simulink model "verify_voltrip_3series"  (R2016a)
settings: Solver=ode4  StartTime=0.0  StopTime=Tmax  FixedStep=Ts  RelTol=1e-3
values from neighbouring files (symbols this model uses):
  Cdc = 50e-6    (= 5e-05)    [pemd_simulink_base.m]
  Lload = Xload/wout    [pemd_simulink_base.m]
  ma = 0.9    [optim_v1.m]    (also in pemd_simulink_base.m = 0.8)
  phase = [0 (k-1)*10 (k-1)*20 (k-1)*30]    [pemd_simulink_base.m]
  Rin = 10    [pemd_simulink_base.m]
  Rload = Zload*pf    [pemd_simulink_base.m]
  Ts = 1e-6    (= 1e-06)    [pemd_simulink_base.m]
  Tth = 0.04    [pemd_simulink_base.m]
  Vin = Vdc + Rin*(Ptotal/Vdc)    (= 697.604412924)    [pemd_simulink_base.m]
  wout = 2*pi*fout    (= 314.159265359)    [pemd_simulink_base.m]
libraries: powerlib x41, powerlib_meascontrol x16, simulink x8
settings Model: Creator=ugurm  LastModifiedBy=mesutto
settings DataIOCC: LimitDataPoints=on  SaveFormat=Array
settings DebuggingCC: UnderspecifiedInitializationDetection=Classic  MergeDetectMultiDrivingBlocksExec=none  SolverPrmCheckMsg=warning  StateNameClashWarn=warning
settings HardwareCC: ProdBitPerPointer=32  ProdLargestAtomicFloat=None  ProdIntDivRoundTo=Undefined  ProdEndianess=Unspecified  ProdWordSize=32  ProdHWDeviceType=32-bit Generic
settings ModelReferenceCC: PropagateSignalLabelsOutOfModel=off
settings ConfigComp: CovModelRefEnable=Off

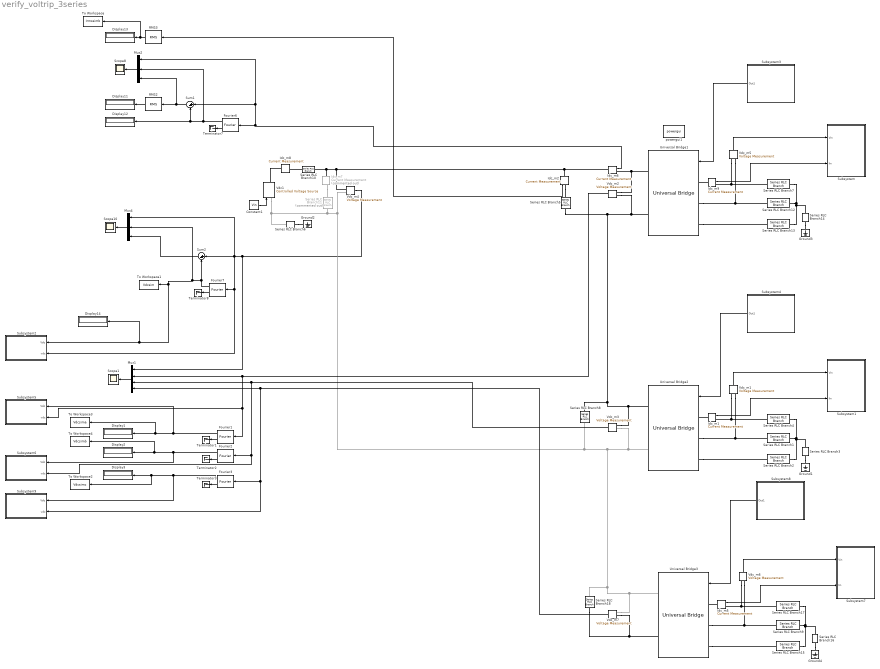
== system verify_voltrip_3series ==
  Constant1 : Constant  Value=Vin
  Display{1..3,11..14} (7 alike) : Display
  Fourier{1..3,7} (4 alike) : powerlib_meascontrol/Measurements/Fourier  Freq=fout  n=0  InInit=[0, 0]  Ts=Ts
  Fourier6 : powerlib_meascontrol/Measurements/Fourier  Freq=fout  n=0  InInit=[20, 0]  Ts=Ts
  Ground{1..4} (4 alike) : powerlib/Elements/Ground  LConnTagsString=a
  Idc_m{1..2,5..6,8..9} (6 alike) : powerlib/Measurements/Current Measurement  PhasorSimulation=off  OutputType=Complex  PSBequivalent=0
  Idc_m7 : powerlib/Measurements/Current Measurement  Commented=on  PhasorSimulation=off  OutputType=Complex  PSBequivalent=0
  Mux1 : Mux
  Mux2 : Mux  Inputs=3
  Mux4 : Mux  Inputs=3
  RMS2 : powerlib_meascontrol/Measurements/RMS  TrueRMS=on  Freq=fout  RMSInit=10  Ts=Ts
  RMS3 : powerlib_meascontrol/Measurements/RMS  TrueRMS=on  Freq=fout  RMSInit=10  Ts=Ts
  Scope1 : Scope
  Scope10 : Scope
  Scope8 : Scope
  Series RLC Branch{1..2,4,7,9,12..13,15,17} (9 alike) : powerlib/Elements/Series RLC Branch  LConnTagsString=__new0  RConnTagsString=__new0  BranchType=RL  Resistance=Rload  Inductance=Lload  SetiL0=off  InitialCurrent=0  Capacitance=1e-6  Setx0=off  InitialVoltage=0  Measurements=None
  Series RLC Branch10 : powerlib/Elements/Series RLC Branch  LConnTagsString=__new0  RConnTagsString=__new0  BranchType=R  Resistance=Rin  Inductance=Lload  SetiL0=off  InitialCurrent=0  Capacitance=1e-6  Setx0=off  InitialVoltage=0  Measurements=None
  Series RLC Branch11 : powerlib/Elements/Series RLC Branch  Commented=on  LConnTagsString=__new0  RConnTagsString=__new0  BranchType=C  Resistance=1e12  Inductance=Lload  SetiL0=off  InitialCurrent=0  Capacitance=Cdc  Setx0=off  InitialVoltage=0  Measurements=None
  Series RLC Branch{3,6,14,16} (4 alike) : powerlib/Elements/Series RLC Branch  LConnTagsString=__new0  RConnTagsString=__new0  BranchType=R  Resistance=1e12  Inductance=Lload  SetiL0=off  InitialCurrent=0  Capacitance=1e-6  Setx0=off  InitialVoltage=0  Measurements=None
  Series RLC Branch18 : powerlib/Elements/Series RLC Branch  LConnTagsString=__new0  RConnTagsString=__new0  BranchType=C  Resistance=1e12  Inductance=Lload  SetiL0=off  InitialCurrent=0  Capacitance=Cdc  Setx0=off  InitialVoltage=0  Measurements=None
  Series RLC Branch5 : powerlib/Elements/Series RLC Branch  LConnTagsString=__new0  RConnTagsString=__new0  BranchType=C  Resistance=1e12  Inductance=Lload  SetiL0=off  InitialCurrent=0  Capacitance=Cdc  Setx0=off  InitialVoltage=0  Measurements=None
  Series RLC Branch8 : powerlib/Elements/Series RLC Branch  LConnTagsString=__new0  RConnTagsString=__new0  BranchType=C  Resistance=1e12  Inductance=Lload  SetiL0=off  InitialCurrent=0  Capacitance=Cdc  Setx0=off  InitialVoltage=0  Measurements=None
  Subsystem : Subsystem
  Subsystem1 : Subsystem
  Subsystem2 : Subsystem
  Subsystem3 : Subsystem
  Subsystem4 : Subsystem
  Subsystem5 : Subsystem
  Subsystem6 : Subsystem
  Subsystem7 : Subsystem
  Subsystem8 : Subsystem
  Subsystem9 : Subsystem
  Sum1 : Sum  Inputs=|+-
  Sum2 : Sum  Inputs=|+-
  Terminator{1..3,7..8} (5 alike) : Terminator
  To Workspace : ToWorkspace  VariableName=Irmssimb  SampleTime=-1
  To Workspace1 : ToWorkspace  VariableName=Vdcsim  SampleTime=-1
  To Workspace2 : ToWorkspace  VariableName=Vdcsimc  SampleTime=-1
  To Workspace3 : ToWorkspace  VariableName=Vdcsima  SampleTime=-1
  To Workspace4 : ToWorkspace  VariableName=Vdcsimb  SampleTime=-1
  Universal Bridge1 : powerlib/Power Electronics/Universal Bridge  Arms=3  SnubberResistance=1e5  SnubberCapacitance=inf  Device=IGBT / Diodes  Ron=1e-6  Lon=0  ForwardVoltages="[  0  0  ]"  ForwardVoltage=0  GTOparameters=[ 10e-6 , 20e-6 ]  IGBTparameters=[ 1e-6 , 2e-6 ]  Measurements=None  Measurements_2=None  converterType=Rectifier
  Universal Bridge2 : powerlib/Power Electronics/Universal Bridge  Arms=3  SnubberResistance=1e5  SnubberCapacitance=inf  Device=IGBT / Diodes  Ron=1e-6  Lon=0  ForwardVoltages="[  0  0  ]"  ForwardVoltage=0  GTOparameters=[ 10e-6 , 20e-6 ]  IGBTparameters=[ 1e-6 , 2e-6 ]  Measurements=None  Measurements_2=None  converterType=Rectifier
  Universal Bridge3 : powerlib/Power Electronics/Universal Bridge  Arms=3  SnubberResistance=1e5  SnubberCapacitance=inf  Device=IGBT / Diodes  Ron=1e-6  Lon=0  ForwardVoltages="[  0  0  ]"  ForwardVoltage=0  GTOparameters=[ 10e-6 , 20e-6 ]  IGBTparameters=[ 1e-6 , 2e-6 ]  Measurements=None  Measurements_2=None  converterType=Rectifier
  Vdc1 : powerlib/Electrical Sources/Controlled Voltage Source  Initialize=off  Source_Type=DC  Amplitude=200  Phase=0  Frequency=0  Measurements=None
  Vdc_m{1..7} (7 alike) : powerlib/Measurements/Voltage Measurement  PhasorSimulation=off  OutputType=Complex  PSBequivalent=0
  powergui1 : powerlib/powergui  Priority=1  SimulationMode=Discrete  SolverType=Tustin  SampleTime=Ts  frequency=60  SPID=off  DisableSnubberDevices=off  DisableRonSwitches=off  DisableVfSwitches=off  SwTol=0  DisplayEquations=off  Interpol=off  ExternalGateDelay=off  methode=off  Ts=0  FunctionMessages=off  echomessages=off  HookPort=off  EnableUseOfTLC=off  x0status=blocks  frequencyindice=0  Pbase=100e6  ErrMax=1e-4  Iterations=50  UnitsV=kV  UnitsW=MW  buscounter=0  RestoreLinks=warning  ResistiveCurrentMeasurement=off  Frange=[0:2:500]  Ylog=off  Xlog=on  ShowGrid=off  save=off  variable=ZData  structure=idc  ZoomFFT=off  StartTime=0.1  cycles=20  DisplayStyle=5  fundamental=50  FreqAxis=off  MaxFrequency=20000  frequencyindicesteady=1  RmsSteady=1  display=off
  wires:
  Fourier6/2 -> Terminator7/1
  RMS2/1 -> Display11/1
  Fourier6/1 -> Mux2/2, Sum1/2, Display12/1
  Sum1/1 -> Mux2/3, RMS2/1
  Constant1/1 -> Vdc1/1
  Idc_m6/1 -> Sum1/1, Mux2/1, Fourier6/1
  Mux2/1 -> Scope8/1
  RMS3/1 -> To Workspace/1, Display13/1
  Fourier7/2 -> Terminator8/1
  Fourier7/1 -> Sum2/2, Mux4/2, Display14/1, Subsystem2/1(Vdc), To Workspace1/1
  Vdc_m4/1 -> Mux1/1, Mux4/1, Subsystem2/2(vdc), Fourier7/1, Sum2/1
  Mux4/1 -> Scope10/1
  Sum2/1 -> Mux4/3
  Subsystem3/1(Out1) -> Universal Bridge1/1
  Vdc_m5/1 -> Subsystem/1(Vin)
  Idc_m9/1 -> Subsystem/2(Iin)
  Subsystem4/1(Out1) -> Universal Bridge2/1
  Vdc_m1/1 -> Subsystem1/1(Vin)
  Idc_m1/1 -> Subsystem1/2(Iin)
  Fourier1/2 -> Terminator1/1
  Fourier1/1 -> Subsystem5/1(Vdc), To Workspace3/1, Display1/1
  Mux1/1 -> Scope1/1
  Fourier2/2 -> Terminator2/1
  Fourier2/1 -> Subsystem6/1(Vdc), Display2/1, To Workspace4/1
  Idc_m2/1 -> RMS3/1
  Subsystem8/1(Out1) -> Universal Bridge3/1
  Vdc_m6/1 -> Subsystem7/1(Vin)
  Idc_m5/1 -> Subsystem7/2(Iin)
  Fourier3/2 -> Terminator3/1
  Fourier3/1 -> Subsystem9/1(Vdc), To Workspace2/1, Display3/1
  Vdc_m2/1 -> Subsystem5/2(vdc), Fourier1/1, Mux1/2
  Vdc_m3/1 -> Subsystem6/2(vdc), Fourier2/1, Mux1/3
  Vdc_m7/1 -> Subsystem9/2(vdc), Fourier3/1, Mux1/4
  connections:
  Universal Bridge1/RConn1 -- Vdc_m2/LConn1 -- Idc_m6/RConn1
  Idc_m7/RConn1 -- Series RLC Branch11/LConn1
  Series RLC Branch6/RConn1 -- Ground2/LConn1
  Series RLC Branch10/RConn1 -- Idc_m8/RConn1
  Vdc1/RConn1 -- Idc_m8/LConn1
  Universal Bridge1/LConn3 -- Series RLC Branch13/LConn1
  Series RLC Branch12/LConn1 -- Universal Bridge1/LConn2 -- Vdc_m5/LConn2
  Vdc_m5/LConn1 -- Idc_m9/RConn1 -- Series RLC Branch7/LConn1
  Series RLC Branch12/RConn1 -- Series RLC Branch14/LConn1 -- Series RLC Branch13/RConn1 -- Series RLC Branch7/RConn1
  Series RLC Branch14/RConn1 -- Ground3/LConn1
  Idc_m9/LConn1 -- Universal Bridge1/LConn1
  Vdc_m1/LConn2 -- Universal Bridge2/LConn2 -- Series RLC Branch1/LConn1
  Vdc_m1/LConn1 -- Idc_m1/RConn1 -- Series RLC Branch4/LConn1
  Series RLC Branch2/RConn1 -- Series RLC Branch4/RConn1 -- Series RLC Branch1/RConn1 -- Series RLC Branch3/LConn1
  Idc_m1/LConn1 -- Universal Bridge2/LConn1
  Series RLC Branch3/RConn1 -- Ground1/LConn1
  Universal Bridge2/LConn3 -- Series RLC Branch2/LConn1
  Idc_m2/RConn1 -- Series RLC Branch5/LConn1
  Vdc_m4/LConn1 -- Idc_m6/LConn1 -- Idc_m2/LConn1 -- Series RLC Branch10/LConn1 -- Idc_m7/LConn1
  Series RLC Branch5/RConn1 -- Series RLC Branch8/LConn1 -- Vdc_m3/LConn1 -- Universal Bridge2/RConn1 -- Vdc_m2/LConn2 -- Universal Bridge1/RConn2
  Vdc_m6/LConn2 -- Universal Bridge3/LConn2 -- Series RLC Branch9/LConn1
  Vdc_m6/LConn1 -- Idc_m5/RConn1 -- Series RLC Branch17/LConn1
  Series RLC Branch15/RConn1 -- Series RLC Branch16/LConn1 -- Series RLC Branch17/RConn1 -- Series RLC Branch9/RConn1
  Universal Bridge3/LConn3 -- Series RLC Branch15/LConn1
  Idc_m5/LConn1 -- Universal Bridge3/LConn1
  Series RLC Branch16/RConn1 -- Ground4/LConn1
  Series RLC Branch11/RConn1 -- Series RLC Branch18/LConn1 -- Vdc_m7/LConn1 -- Universal Bridge3/RConn1 -- Vdc_m3/LConn2 -- Universal Bridge2/RConn2 -- Series RLC Branch8/RConn1 -- Vdc_m4/LConn2 -- Vdc1/LConn1 -- Series RLC Branch6/LConn1
  Vdc_m7/LConn2 -- Series RLC Branch18/RConn1 -- Universal Bridge3/RConn2

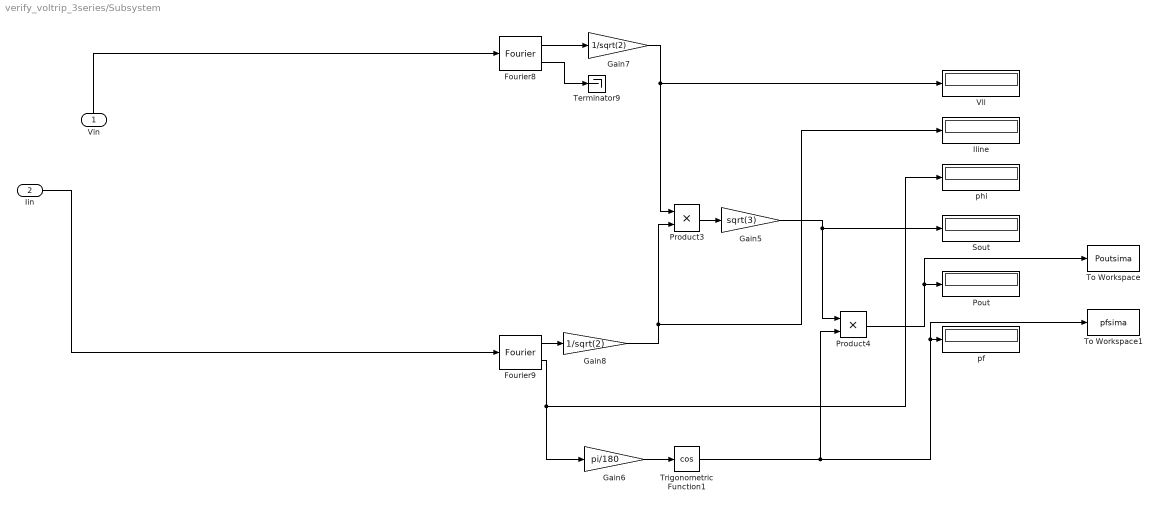
== system verify_voltrip_3series/Subsystem ==
  Vin : Inport
  Iin : Inport  Port=2
  Fourier8 : powerlib_meascontrol/Measurements/Fourier  Freq=fout  n=1  InInit=[0, 0]  Ts=Ts
  Fourier9 : powerlib_meascontrol/Measurements/Fourier  Freq=fout  n=1  InInit=[0, 0]  Ts=Ts
  Gain5 : Gain  Gain=sqrt(3)
  Gain6 : Gain  Gain=pi/180
  Gain7 : Gain  Gain=1/sqrt(2)
  Gain8 : Gain  Gain=1/sqrt(2)
  Iline : Display
  Pout : Display
  Product3 : Product
  Product4 : Product
  Sout : Display
      settings: Format=short_e
  Terminator9 : Terminator
  To Workspace : ToWorkspace  VariableName=Poutsima  SampleTime=-1
  To Workspace1 : ToWorkspace  VariableName=pfsima  SampleTime=-1
  Trigonometric Function1 : Trigonometry  Operator=cos
  Vll : Display
  pf : Display
  phi : Display
  wires:
  Gain6/1 -> Trigonometric Function1/1
  Gain8/1 -> Iline/1, Product3/2
  Gain5/1 -> Product4/1, Sout/1
  Trigonometric Function1/1 -> Product4/2, To Workspace1/1, pf/1
  Vin/1 -> Fourier8/1
  Iin/1 -> Fourier9/1
  Fourier8/2 -> Terminator9/1
  Fourier8/1 -> Gain7/1
  Product3/1 -> Gain5/1
  Gain7/1 -> Product3/1, Vll/1
  Product4/1 -> To Workspace/1, Pout/1
  Fourier9/2 -> Gain6/1, phi/1
  Fourier9/1 -> Gain8/1

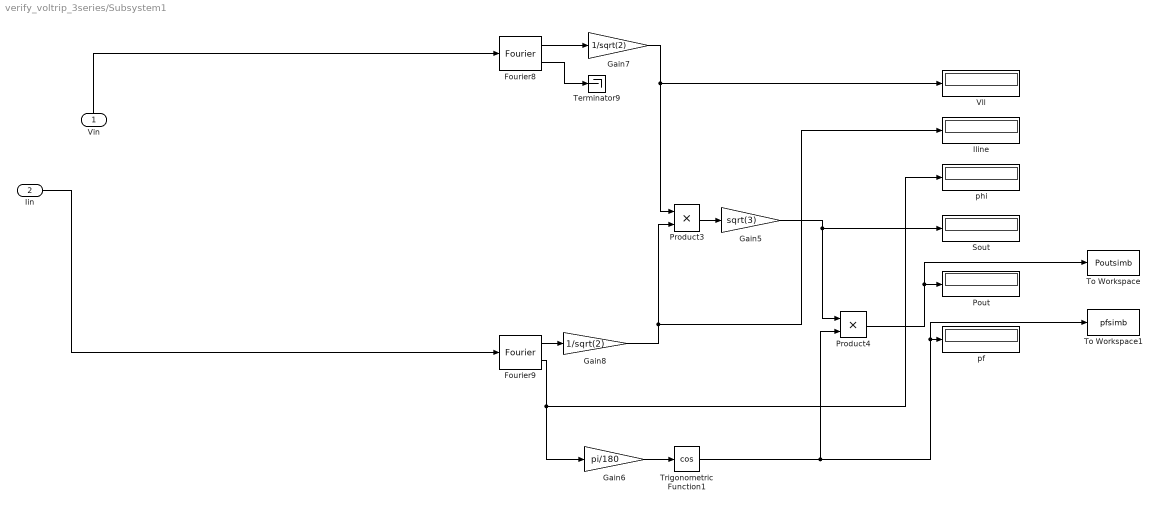
== system verify_voltrip_3series/Subsystem1 ==
  Vin : Inport
  Iin : Inport  Port=2
  Fourier8 : powerlib_meascontrol/Measurements/Fourier  Freq=fout  n=1  InInit=[0, 0]  Ts=Ts
  Fourier9 : powerlib_meascontrol/Measurements/Fourier  Freq=fout  n=1  InInit=[0, 0]  Ts=Ts
  Gain5 : Gain  Gain=sqrt(3)
  Gain6 : Gain  Gain=pi/180
  Gain7 : Gain  Gain=1/sqrt(2)
  Gain8 : Gain  Gain=1/sqrt(2)
  Iline : Display
  Pout : Display
  Product3 : Product
  Product4 : Product
  Sout : Display
      settings: Format=short_e
  Terminator9 : Terminator
  To Workspace : ToWorkspace  VariableName=Poutsimb  SampleTime=-1
  To Workspace1 : ToWorkspace  VariableName=pfsimb  SampleTime=-1
  Trigonometric Function1 : Trigonometry  Operator=cos
  Vll : Display
  pf : Display
  phi : Display
  wires:
  Gain6/1 -> Trigonometric Function1/1
  Gain8/1 -> Iline/1, Product3/2
  Gain5/1 -> Product4/1, Sout/1
  Trigonometric Function1/1 -> Product4/2, To Workspace1/1, pf/1
  Vin/1 -> Fourier8/1
  Iin/1 -> Fourier9/1
  Fourier8/2 -> Terminator9/1
  Fourier8/1 -> Gain7/1
  Product3/1 -> Gain5/1
  Gain7/1 -> Product3/1, Vll/1
  Product4/1 -> To Workspace/1, Pout/1
  Fourier9/2 -> Gain6/1, phi/1
  Fourier9/1 -> Gain8/1

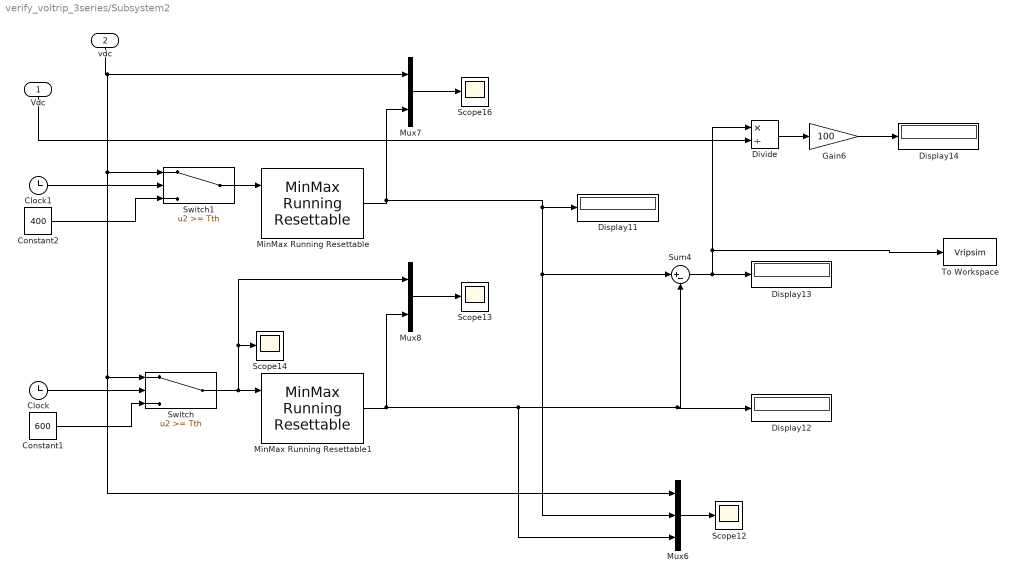
== system verify_voltrip_3series/Subsystem2 ==
  Vdc : Inport
  vdc : Inport  Port=2
  Clock : Clock
  Clock1 : Clock
  Constant1 : Constant  Value=600  SampleTime=Ts
  Constant2 : Constant  Value=400  SampleTime=Ts
  Display{11..14} (4 alike) : Display
  Divide : Product  Inputs=*/
  Gain6 : Gain  Gain=100
  MinMax Running Resettable : simulink/Math Operations/MinMax Running Resettable  Function=max  vinit=400
  MinMax Running Resettable1 : simulink/Math Operations/MinMax Running Resettable  Function=min  vinit=600
  Mux6 : Mux  Inputs=3
  Mux7 : Mux  Inputs=2
  Mux8 : Mux  Inputs=2
  Scope{12..14,16} (4 alike) : Scope
  Sum4 : Sum  Inputs=|+-
  Switch : Switch  Threshold=Tth
  Switch1 : Switch  Threshold=Tth
  To Workspace : ToWorkspace  VariableName=Vripsim  SampleTime=-1
  wires:
  MinMax Running Resettable/1 -> Display11/1, Mux6/2, Sum4/1, Mux7/2
  Clock/1 -> Switch/2
  Mux8/1 -> Scope13/1
  Gain6/1 -> Display14/1
  Constant1/1 -> Switch/3
  MinMax Running Resettable1/1 -> Mux6/3, Display12/1, Sum4/2, Mux8/2
  Mux7/1 -> Scope16/1
  Switch/1 -> Mux8/1, Scope14/1, MinMax Running Resettable1/1
  Divide/1 -> Gain6/1
  Mux6/1 -> Scope12/1
  Vdc/1 -> Divide/2
  vdc/1 -> Mux7/1, Switch1/1, Mux6/1, Switch/1
  Clock1/1 -> Switch1/2
  Constant2/1 -> Switch1/3
  Switch1/1 -> MinMax Running Resettable/1
  Sum4/1 -> To Workspace/1, Divide/1, Display13/1

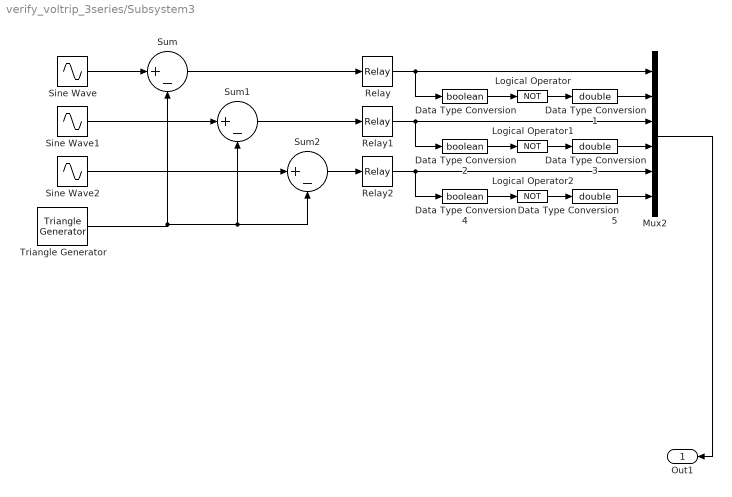
== system verify_voltrip_3series/Subsystem3 ==
  Data Type Conversion : DataTypeConversion  OutDataTypeStr=boolean
  Data Type Conversion1 : DataTypeConversion  OutDataTypeStr=double
  Data Type Conversion2 : DataTypeConversion  OutDataTypeStr=boolean
  Data Type Conversion3 : DataTypeConversion  OutDataTypeStr=double
  Data Type Conversion4 : DataTypeConversion  OutDataTypeStr=boolean
  Data Type Conversion5 : DataTypeConversion  OutDataTypeStr=double
  Logical Operator : Logic  Operator=NOT  AllPortsSameDT=off  OutDataTypeStr=boolean
  Logical Operator1 : Logic  Operator=NOT  AllPortsSameDT=off  OutDataTypeStr=boolean
  Logical Operator2 : Logic  Operator=NOT  AllPortsSameDT=off  OutDataTypeStr=boolean
  Mux2 : Mux  Inputs=6
  Relay : Relay
  Relay1 : Relay
  Relay2 : Relay
  Sine Wave : Sin  Amplitude=ma  Frequency=wout  SampleTime=0
  Sine Wave1 : Sin  Amplitude=ma  Frequency=wout  Phase=-2*pi/3  SampleTime=0
  Sine Wave2 : Sin  Amplitude=ma  Frequency=wout  Phase=2*pi/3  SampleTime=0
  Sum : Sum  Inputs=|+-
  Sum1 : Sum  Inputs=|+-
  Sum2 : Sum  Inputs=|+-
  Triangle Generator : powerlib_meascontrol/Pulse & Signal Generators/Triangle Generator  Freq=fsw  Phase=phase(1)  Ts=Ts
  Out1 : Outport
  wires:
  Logical Operator1/1 -> Data Type Conversion3/1
  Sum/1 -> Relay/1
  Triangle Generator/1 -> Sum1/2, Sum2/2, Sum/2
  Logical Operator/1 -> Data Type Conversion1/1
  Relay1/1 -> Data Type Conversion2/1, Mux2/3
  Logical Operator2/1 -> Data Type Conversion5/1
  Data Type Conversion4/1 -> Logical Operator2/1
  Data Type Conversion2/1 -> Logical Operator1/1
  Data Type Conversion5/1 -> Mux2/6
  Sine Wave2/1 -> Sum2/1
  Data Type Conversion3/1 -> Mux2/4
  Sum1/1 -> Relay1/1
  Relay2/1 -> Data Type Conversion4/1, Mux2/5
  Relay/1 -> Data Type Conversion/1, Mux2/1
  Mux2/1 -> Out1/1
  Data Type Conversion1/1 -> Mux2/2
  Sine Wave/1 -> Sum/1
  Sine Wave1/1 -> Sum1/1
  Data Type Conversion/1 -> Logical Operator/1
  Sum2/1 -> Relay2/1

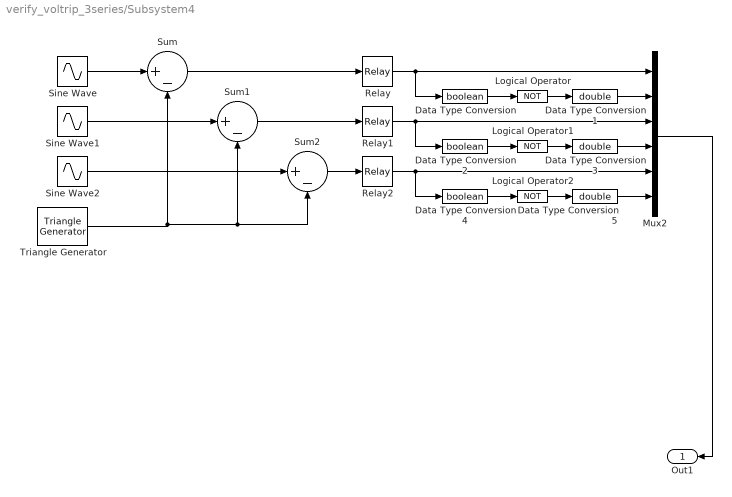
== system verify_voltrip_3series/Subsystem4 ==
  Data Type Conversion : DataTypeConversion  OutDataTypeStr=boolean
  Data Type Conversion1 : DataTypeConversion  OutDataTypeStr=double
  Data Type Conversion2 : DataTypeConversion  OutDataTypeStr=boolean
  Data Type Conversion3 : DataTypeConversion  OutDataTypeStr=double
  Data Type Conversion4 : DataTypeConversion  OutDataTypeStr=boolean
  Data Type Conversion5 : DataTypeConversion  OutDataTypeStr=double
  Logical Operator : Logic  Operator=NOT  AllPortsSameDT=off  OutDataTypeStr=boolean
  Logical Operator1 : Logic  Operator=NOT  AllPortsSameDT=off  OutDataTypeStr=boolean
  Logical Operator2 : Logic  Operator=NOT  AllPortsSameDT=off  OutDataTypeStr=boolean
  Mux2 : Mux  Inputs=6
  Relay : Relay
  Relay1 : Relay
  Relay2 : Relay
  Sine Wave : Sin  Amplitude=ma  Frequency=wout  SampleTime=0
  Sine Wave1 : Sin  Amplitude=ma  Frequency=wout  Phase=-2*pi/3  SampleTime=0
  Sine Wave2 : Sin  Amplitude=ma  Frequency=wout  Phase=2*pi/3  SampleTime=0
  Sum : Sum  Inputs=|+-
  Sum1 : Sum  Inputs=|+-
  Sum2 : Sum  Inputs=|+-
  Triangle Generator : powerlib_meascontrol/Pulse & Signal Generators/Triangle Generator  Freq=fsw  Phase=phase(2)  Ts=Ts
  Out1 : Outport
  wires:
  Logical Operator1/1 -> Data Type Conversion3/1
  Sum/1 -> Relay/1
  Triangle Generator/1 -> Sum1/2, Sum2/2, Sum/2
  Logical Operator/1 -> Data Type Conversion1/1
  Relay1/1 -> Data Type Conversion2/1, Mux2/3
  Logical Operator2/1 -> Data Type Conversion5/1
  Data Type Conversion4/1 -> Logical Operator2/1
  Data Type Conversion2/1 -> Logical Operator1/1
  Data Type Conversion5/1 -> Mux2/6
  Sine Wave2/1 -> Sum2/1
  Data Type Conversion3/1 -> Mux2/4
  Sum1/1 -> Relay1/1
  Relay2/1 -> Data Type Conversion4/1, Mux2/5
  Relay/1 -> Data Type Conversion/1, Mux2/1
  Mux2/1 -> Out1/1
  Data Type Conversion1/1 -> Mux2/2
  Sine Wave/1 -> Sum/1
  Sine Wave1/1 -> Sum1/1
  Data Type Conversion/1 -> Logical Operator/1
  Sum2/1 -> Relay2/1

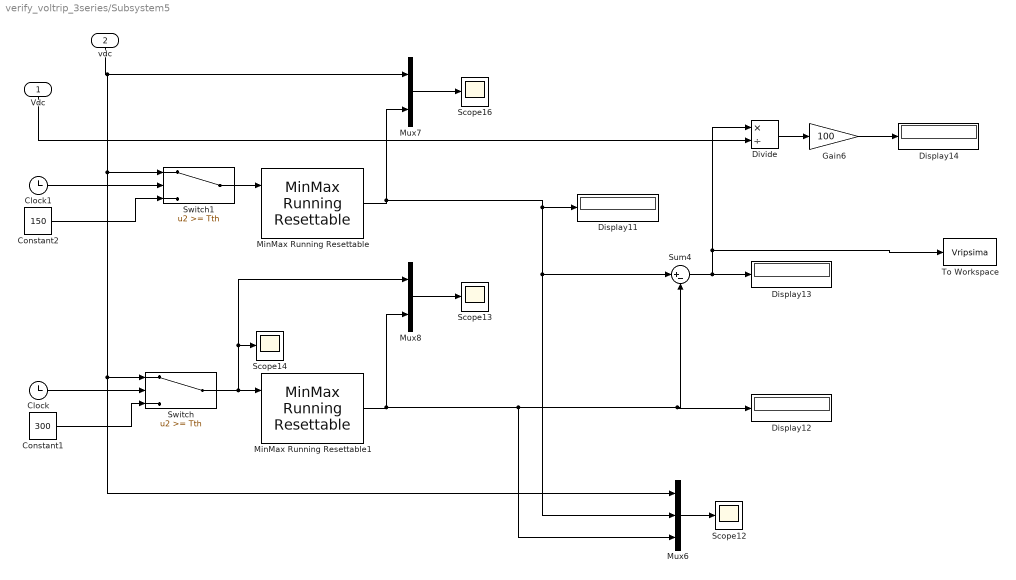
== system verify_voltrip_3series/Subsystem5 ==
  Vdc : Inport
  vdc : Inport  Port=2
  Clock : Clock
  Clock1 : Clock
  Constant1 : Constant  Value=300  SampleTime=Ts
  Constant2 : Constant  Value=150  SampleTime=Ts
  Display{11..14} (4 alike) : Display
  Divide : Product  Inputs=*/
  Gain6 : Gain  Gain=100
  MinMax Running Resettable : simulink/Math Operations/MinMax Running Resettable  Function=max  vinit=150
  MinMax Running Resettable1 : simulink/Math Operations/MinMax Running Resettable  Function=min  vinit=300
  Mux6 : Mux  Inputs=3
  Mux7 : Mux  Inputs=2
  Mux8 : Mux  Inputs=2
  Scope{12..14,16} (4 alike) : Scope
  Sum4 : Sum  Inputs=|+-
  Switch : Switch  Threshold=Tth
  Switch1 : Switch  Threshold=Tth
  To Workspace : ToWorkspace  VariableName=Vripsima  SampleTime=-1
  wires:
  MinMax Running Resettable/1 -> Display11/1, Mux6/2, Sum4/1, Mux7/2
  Clock/1 -> Switch/2
  Mux8/1 -> Scope13/1
  Gain6/1 -> Display14/1
  Constant1/1 -> Switch/3
  MinMax Running Resettable1/1 -> Mux6/3, Display12/1, Sum4/2, Mux8/2
  Mux7/1 -> Scope16/1
  Switch/1 -> Mux8/1, Scope14/1, MinMax Running Resettable1/1
  Divide/1 -> Gain6/1
  Mux6/1 -> Scope12/1
  Vdc/1 -> Divide/2
  vdc/1 -> Mux7/1, Switch1/1, Mux6/1, Switch/1
  Clock1/1 -> Switch1/2
  Constant2/1 -> Switch1/3
  Switch1/1 -> MinMax Running Resettable/1
  Sum4/1 -> To Workspace/1, Divide/1, Display13/1

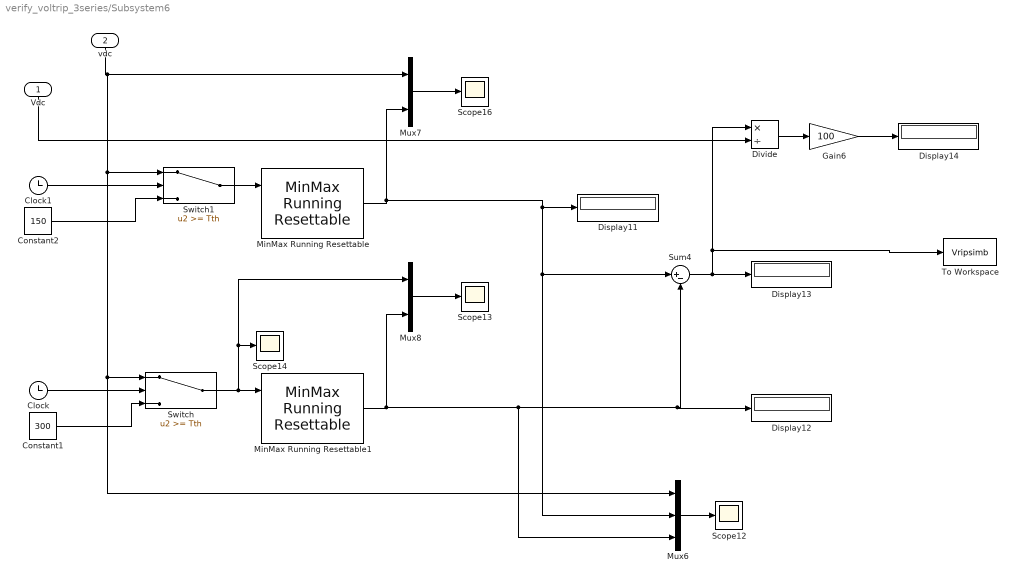
== system verify_voltrip_3series/Subsystem6 ==
  Vdc : Inport
  vdc : Inport  Port=2
  Clock : Clock
  Clock1 : Clock
  Constant1 : Constant  Value=300  SampleTime=Ts
  Constant2 : Constant  Value=150  SampleTime=Ts
  Display{11..14} (4 alike) : Display
  Divide : Product  Inputs=*/
  Gain6 : Gain  Gain=100
  MinMax Running Resettable : simulink/Math Operations/MinMax Running Resettable  Function=max  vinit=150
  MinMax Running Resettable1 : simulink/Math Operations/MinMax Running Resettable  Function=min  vinit=300
  Mux6 : Mux  Inputs=3
  Mux7 : Mux  Inputs=2
  Mux8 : Mux  Inputs=2
  Scope{12..14,16} (4 alike) : Scope
  Sum4 : Sum  Inputs=|+-
  Switch : Switch  Threshold=Tth
  Switch1 : Switch  Threshold=Tth
  To Workspace : ToWorkspace  VariableName=Vripsimb  SampleTime=-1
  wires:
  MinMax Running Resettable/1 -> Display11/1, Mux6/2, Sum4/1, Mux7/2
  Clock/1 -> Switch/2
  Mux8/1 -> Scope13/1
  Gain6/1 -> Display14/1
  Constant1/1 -> Switch/3
  MinMax Running Resettable1/1 -> Mux6/3, Display12/1, Sum4/2, Mux8/2
  Mux7/1 -> Scope16/1
  Switch/1 -> Mux8/1, Scope14/1, MinMax Running Resettable1/1
  Divide/1 -> Gain6/1
  Mux6/1 -> Scope12/1
  Vdc/1 -> Divide/2
  vdc/1 -> Mux7/1, Switch1/1, Mux6/1, Switch/1
  Clock1/1 -> Switch1/2
  Constant2/1 -> Switch1/3
  Switch1/1 -> MinMax Running Resettable/1
  Sum4/1 -> To Workspace/1, Divide/1, Display13/1

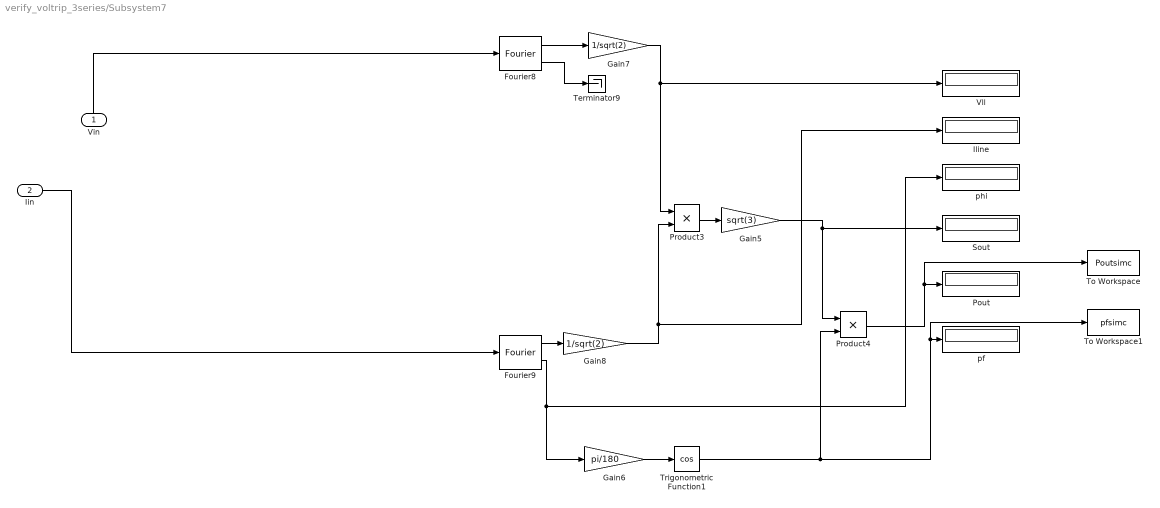
== system verify_voltrip_3series/Subsystem7 ==
  Vin : Inport
  Iin : Inport  Port=2
  Fourier8 : powerlib_meascontrol/Measurements/Fourier  Freq=fout  n=1  InInit=[0, 0]  Ts=Ts
  Fourier9 : powerlib_meascontrol/Measurements/Fourier  Freq=fout  n=1  InInit=[0, 0]  Ts=Ts
  Gain5 : Gain  Gain=sqrt(3)
  Gain6 : Gain  Gain=pi/180
  Gain7 : Gain  Gain=1/sqrt(2)
  Gain8 : Gain  Gain=1/sqrt(2)
  Iline : Display
  Pout : Display
  Product3 : Product
  Product4 : Product
  Sout : Display
      settings: Format=short_e
  Terminator9 : Terminator
  To Workspace : ToWorkspace  VariableName=Poutsimc  SampleTime=-1
  To Workspace1 : ToWorkspace  VariableName=pfsimc  SampleTime=-1
  Trigonometric Function1 : Trigonometry  Operator=cos
  Vll : Display
  pf : Display
  phi : Display
  wires:
  Gain6/1 -> Trigonometric Function1/1
  Gain8/1 -> Iline/1, Product3/2
  Gain5/1 -> Product4/1, Sout/1
  Trigonometric Function1/1 -> Product4/2, To Workspace1/1, pf/1
  Vin/1 -> Fourier8/1
  Iin/1 -> Fourier9/1
  Fourier8/2 -> Terminator9/1
  Fourier8/1 -> Gain7/1
  Product3/1 -> Gain5/1
  Gain7/1 -> Product3/1, Vll/1
  Product4/1 -> To Workspace/1, Pout/1
  Fourier9/2 -> Gain6/1, phi/1
  Fourier9/1 -> Gain8/1

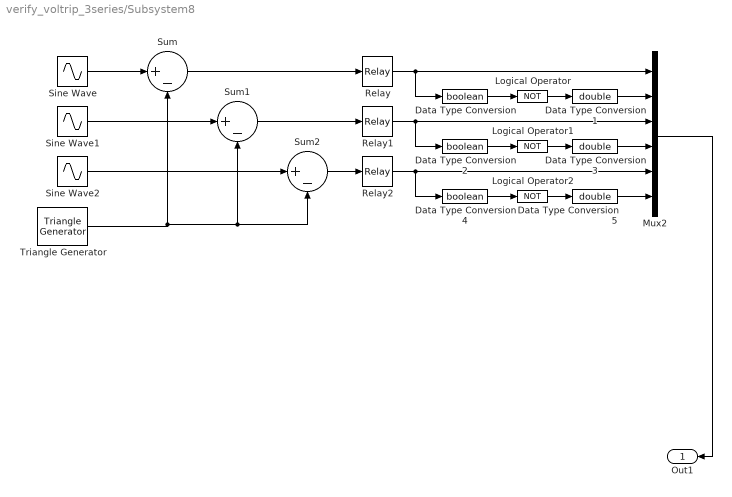
== system verify_voltrip_3series/Subsystem8 ==
  Data Type Conversion : DataTypeConversion  OutDataTypeStr=boolean
  Data Type Conversion1 : DataTypeConversion  OutDataTypeStr=double
  Data Type Conversion2 : DataTypeConversion  OutDataTypeStr=boolean
  Data Type Conversion3 : DataTypeConversion  OutDataTypeStr=double
  Data Type Conversion4 : DataTypeConversion  OutDataTypeStr=boolean
  Data Type Conversion5 : DataTypeConversion  OutDataTypeStr=double
  Logical Operator : Logic  Operator=NOT  AllPortsSameDT=off  OutDataTypeStr=boolean
  Logical Operator1 : Logic  Operator=NOT  AllPortsSameDT=off  OutDataTypeStr=boolean
  Logical Operator2 : Logic  Operator=NOT  AllPortsSameDT=off  OutDataTypeStr=boolean
  Mux2 : Mux  Inputs=6
  Relay : Relay
  Relay1 : Relay
  Relay2 : Relay
  Sine Wave : Sin  Amplitude=ma  Frequency=wout  SampleTime=0
  Sine Wave1 : Sin  Amplitude=ma  Frequency=wout  Phase=-2*pi/3  SampleTime=0
  Sine Wave2 : Sin  Amplitude=ma  Frequency=wout  Phase=2*pi/3  SampleTime=0
  Sum : Sum  Inputs=|+-
  Sum1 : Sum  Inputs=|+-
  Sum2 : Sum  Inputs=|+-
  Triangle Generator : powerlib_meascontrol/Pulse & Signal Generators/Triangle Generator  Freq=fsw  Phase=phase(3)  Ts=Ts
  Out1 : Outport
  wires:
  Logical Operator1/1 -> Data Type Conversion3/1
  Sum/1 -> Relay/1
  Triangle Generator/1 -> Sum1/2, Sum2/2, Sum/2
  Logical Operator/1 -> Data Type Conversion1/1
  Relay1/1 -> Data Type Conversion2/1, Mux2/3
  Logical Operator2/1 -> Data Type Conversion5/1
  Data Type Conversion4/1 -> Logical Operator2/1
  Data Type Conversion2/1 -> Logical Operator1/1
  Data Type Conversion5/1 -> Mux2/6
  Sine Wave2/1 -> Sum2/1
  Data Type Conversion3/1 -> Mux2/4
  Sum1/1 -> Relay1/1
  Relay2/1 -> Data Type Conversion4/1, Mux2/5
  Relay/1 -> Data Type Conversion/1, Mux2/1
  Mux2/1 -> Out1/1
  Data Type Conversion1/1 -> Mux2/2
  Sine Wave/1 -> Sum/1
  Sine Wave1/1 -> Sum1/1
  Data Type Conversion/1 -> Logical Operator/1
  Sum2/1 -> Relay2/1

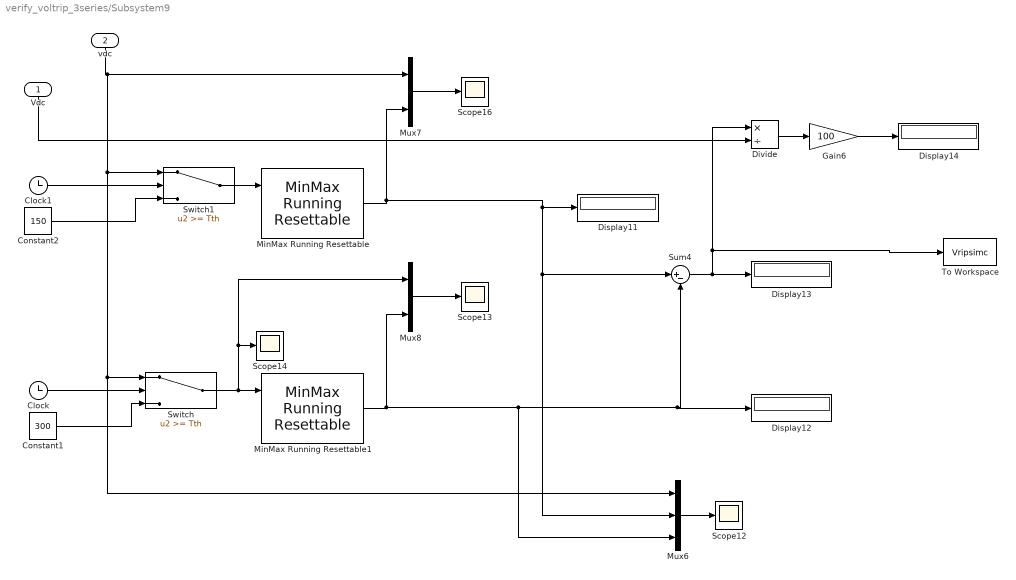
== system verify_voltrip_3series/Subsystem9 ==
  Vdc : Inport
  vdc : Inport  Port=2
  Clock : Clock
  Clock1 : Clock
  Constant1 : Constant  Value=300  SampleTime=Ts
  Constant2 : Constant  Value=150  SampleTime=Ts
  Display{11..14} (4 alike) : Display
  Divide : Product  Inputs=*/
  Gain6 : Gain  Gain=100
  MinMax Running Resettable : simulink/Math Operations/MinMax Running Resettable  Function=max  vinit=150
  MinMax Running Resettable1 : simulink/Math Operations/MinMax Running Resettable  Function=min  vinit=300
  Mux6 : Mux  Inputs=3
  Mux7 : Mux  Inputs=2
  Mux8 : Mux  Inputs=2
  Scope{12..14,16} (4 alike) : Scope
  Sum4 : Sum  Inputs=|+-
  Switch : Switch  Threshold=Tth
  Switch1 : Switch  Threshold=Tth
  To Workspace : ToWorkspace  VariableName=Vripsimc  SampleTime=-1
  wires:
  MinMax Running Resettable/1 -> Display11/1, Mux6/2, Sum4/1, Mux7/2
  Clock/1 -> Switch/2
  Mux8/1 -> Scope13/1
  Gain6/1 -> Display14/1
  Constant1/1 -> Switch/3
  MinMax Running Resettable1/1 -> Mux6/3, Display12/1, Sum4/2, Mux8/2
  Mux7/1 -> Scope16/1
  Switch/1 -> Mux8/1, Scope14/1, MinMax Running Resettable1/1
  Divide/1 -> Gain6/1
  Mux6/1 -> Scope12/1
  Vdc/1 -> Divide/2
  vdc/1 -> Mux7/1, Switch1/1, Mux6/1, Switch/1
  Clock1/1 -> Switch1/2
  Constant2/1 -> Switch1/3
  Switch1/1 -> MinMax Running Resettable/1
  Sum4/1 -> To Workspace/1, Divide/1, Display13/1
